simulink model "HDL_DUC"  (R2025a)
settings: Solver=VariableStepAuto  StartTime=0.0  StopTime=sample_period*512*150  RelTol=1e-3
PreLoadFcn:
  | sample_period=1/800e6;
  | dds=80e6; % ddfs frequency
InitFcn:
  | sample_period=1/800e6;
  | dds=80e6; % ddfs frequency
undefined symbols (not defined in the file): A, A2, B, D, PCIN, S, vsva2197, xcvc1902
libraries: hdlBasic x26, hdlDSPIP x5, dspmlti4 x4, simulink x2, vmcUtilities x1
settings Model: Creator=mmi  LastModifiedBy=robg
settings DebuggingCC: ParameterOverflowMsg=warning  UnconnectedInputMsg=warning  UnconnectedOutputMsg=warning  UnconnectedLineMsg=warning
settings HardwareCC: ProdBitPerPointer=32.0  ProdBitPerSizeT=32.0  ProdBitPerPtrDiffT=32.0  ProdLargestAtomicFloat=None  ProdIntDivRoundTo=Undefined  ProdEndianess=Unspecified  ProdWordSize=32.0  ProdHWDeviceType=ASIC/FPGA->ASIC/FPGA  TargetBitPerLong=64.0  TargetBitPerPointer=64.0  TargetBitPerSizeT=64.0  TargetBitPerPtrDiffT=64.0  TargetLongLongMode=on  TargetIntDivRoundTo=Zero  TargetEndianess=LittleEndian  TargetWordSize=64.0  TargetHWDeviceType=Custom Processor->MATLAB Host Computer  ProdEqTarget=off
settings ModelReferenceCC: EnableRefExpFcnMdlSchedulingChecks=on
settings RTWCC: GPUComputeCapability=3.5  DLArmComputeVersion=19.05

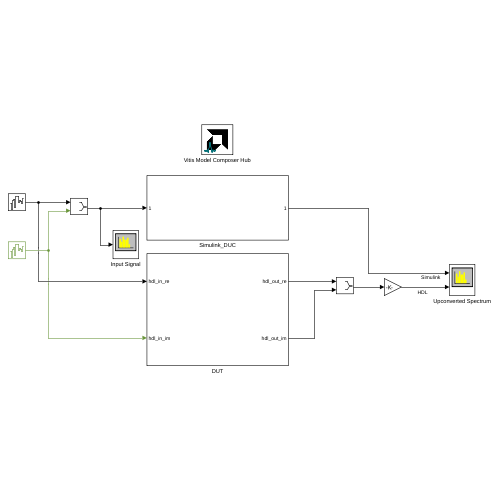
[thumbnail: Simulink's stored preview of the top-level diagram]
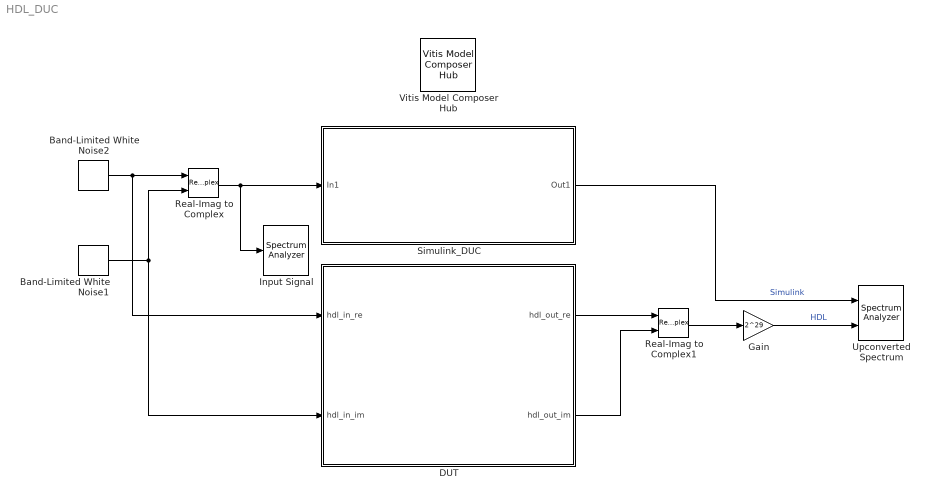
== system HDL_DUC ==
  Band-Limited White Noise1 : simulink/Sources/Band-Limited White Noise  Cov=[0.1]  Ts=sample_period*16  seed=[1]
  Band-Limited White Noise2 : simulink/Sources/Band-Limited White Noise  Cov=[0.1]  Ts=sample_period*16  seed=[2]
  DUT : Subsystem
  Gain : Gain  Gain=2^29  OutDataTypeStr=double
  Input Signal : SpectrumAnalyzer  WindowPosition=[540.000000,419.000000,800.000000,500.000000,]  Visible=on  ScopeFrameLocation=window  Span=50000000  StartFrequency=-25000000  StopFrequency=25000000  YLimits=[22.9484,84.9753]
  Real-Imag to Complex : RealImagToComplex
  Real-Imag to Complex1 : RealImagToComplex
  Simulink_DUC : Subsystem
  Upconverted Spectrum : SpectrumAnalyzer  NumInputPorts=2  WindowPosition=[1096.000000,482.000000,820.000000,457.000000,]  Visible=on  ScopeFrameLocation=window  SampleRate=400000000  AxesScaling=Manual  Span=800000000  StartFrequency=-400000000  StopFrequency=400000000  AveragingMethod=Exponential  YLimits=[63.6592,220.2056]  ShowLegend=on  AllowFFTLengthLessThanSamplesPerUpdate=on
  Vitis Model Composer Hub : vmcUtilities/Vitis Model Composer Hub  Tag=genX  CodeGeneration=off  SubsystemName=DUT  BlockHierPath=HDL_DUC/DUT  CompilationType=HDLCompilation  SubsystemType=HDLNode  ExportTypeV2=IP Catalog  StartColumn=1  NumberOfColumns=1  TargetDirectory=./netlist  exportDesign=on  analyzeDesign=off  validateDesignOnHw=off  ExportType=AI Engines  IpVendor=xilinx.com  IpLibrary=hls  IpVersion=1.0  IpHWLanguage=Verilog  AieCompilerOptions={}  AieSimulatorOptions={}  CreateTestbench=off  TestbenchStackSize=10  RunRtlSim=off  RunCSim=off  RunAieSim=on  enableSimulationTimeout=on  enableGraphIterations=on  AieSimTimeout=50000  AieGraphIterations=-1  RunAieSimProfiling=off  LaunchVitisAnalyzer=on  PlotOutput=off  RunX86Sim=off  X86SimTimeout=10  GenHwImage=off  GenLibadfXo=on  GenHwValidationCode=off  PlatformType=Not Specified  HwSystemType=Baremetal  HwValidationTarget=hw  ProjDevice=xcvc1902-vsva2197-1LP-e-S  ProjDevicePart=xcvc1902-vsva2197-1LP-e-S  AIEType=AIE  SamplePeriod=-1  ClockFrequency=200  DataPathParallelism=1  xilinxfamily=versalaicore  part=xcvc1902  speed=-1LP-e-S  package=vsva2197  directory=./netlist/ip/DUT/src  testbench=off  incr_netlist=off  synthesis_tool=Vivado  clock_wrapper=Clock Enables  dbl_ovrd=According to Block Masks  dcm_input_clock_period=10  sysclk_period=1.25  simulink_period=sample_period  eval_field=0  IPInfoJsonString="{\"DUTSubsystemName\":\"DUT\",\"HDLSubsystem\":{\"SubsystemName\":\"DUT\",\"IPName\":\"HDL_DUC\",\"IPLibrary\":\"VMC\",\"IPVendor\":\"User Company\",\"IPVersion\":\"1.0\",\"TargetDirectory\":\"./netlist\",\"SubsystemDir\":\"./netlist/ip/DUT\",\"FreqHz\":\"800000000\"},\"SubsystemTag\":\"HDLNode\"}"  LogFileName=/proj/xhdhdstaff5/sdegala/Head1/HEAD/VMC_2025_2_July/Examples/HDL/Digital_Filtering/HDL_DUC/netlist/model_composer.log  NThreads=4  IPConfigFile=/tmp/vmctmp-4932002476335468914/HDL_DUC_ipconfig.json
  wires:
  DUT/1(hdl_out_re) -> Real-Imag to Complex1/1
  Simulink_DUC/1(Out1) -> Upconverted Spectrum/1  "Simulink"
  DUT/2(hdl_out_im) -> Real-Imag to Complex1/2
  Real-Imag to Complex1/1 -> Gain/1
  Band-Limited White Noise2/1 -> DUT/1(hdl_in_re), Real-Imag to Complex/1
  Real-Imag to Complex/1 -> Input Signal/1, Simulink_DUC/1(In1)
  Band-Limited White Noise1/1 -> Real-Imag to Complex/2, DUT/2(hdl_in_im)
  Gain/1 -> Upconverted Spectrum/2  "HDL"

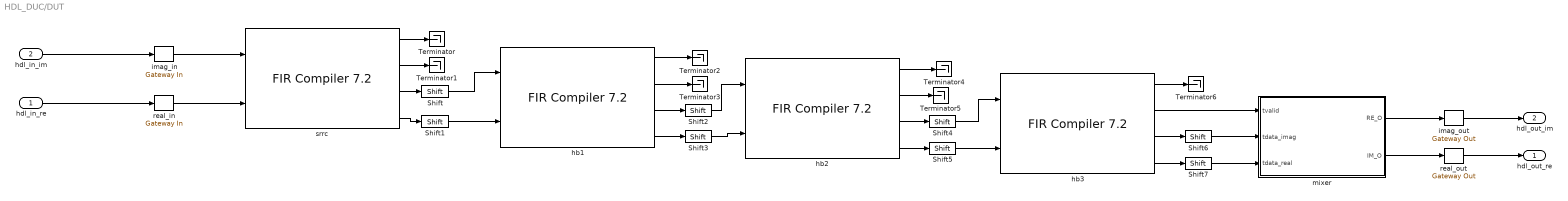
== system HDL_DUC/DUT ==
  hdl_in_re : Inport
  hdl_in_im : Inport  Port=2
  Shift{,1..5} (6 alike) : hdlBasic/Shift  shift_dir=Left  shift_bits=1  en=off  latency=0  precision=Full  arith_type="Signed  (2's comp)"  n_bits=16  bin_pt=14  quantization=Truncate  overflow=Wrap  XmcBlockStatus=1  maskContainerNames=group2  block_type=shift  block_config=sysgen:Shift_config
  Shift6 : hdlBasic/Shift  shift_dir=Left  shift_bits=1  en=off  latency=0  precision=User Defined  arith_type="Signed  (2's comp)"  n_bits=34  bin_pt=0  quantization=Truncate  overflow=Wrap  XmcBlockStatus=1  maskContainerNames=group2  block_type=shift  block_config=sysgen:Shift_config
  Shift7 : hdlBasic/Shift  shift_dir=Left  shift_bits=1  en=off  latency=0  precision=User Defined  arith_type="Signed  (2's comp)"  n_bits=34  bin_pt=0  quantization=Truncate  overflow=Wrap  XmcBlockStatus=1  maskContainerNames=group2  block_type=shift  block_config=sysgen:Shift_config
  Terminator{,1..6} (7 alike) : Terminator
  hb1 : hdlDSPIP/FIR Compiler 7.2   datacoefficienttype=Real  coefficientvector=|  coefficient_sets=1  coefficient_reload=off  filter_type=Interpolation  rate_change_type=Integer  interpolation_rate=2  decimation_rate=1  zero_pack_factor=1  channel_sequence=Basic  number_channels=1  pattern_list='P4-0,P4-1,P4-2,P4-3,P4-4'  number_paths=2  ratespecification=Maximum_Possible  sampleperiod=1  hardwareoversamplingrate=1  coefficient_sign=Signed  quantization=Maximize_Dynamic_Range  coefficient_width=17  bestprecision=on  coefficient_fractional_bits=17  coefficient_structure=Inferred  output_rounding_mode=Truncate_LSBs  output_width=17  filter_architecture=Systolic_Multiply_Accumulate  optimization_goal=Area  optimization_list='None'  data_buffer_type=Automatic  coefficient_buffer_type=Automatic  input_buffer_type=Automatic  output_buffer_type=Automatic  preference_for_other_storage=Automatic  multi_column_support=Automatic  columnconfig='3'  inter_column_pipe_length=4  data_has_tlast=Not_Required  m_data_has_tready=off  s_data_has_fifo=off  s_data_has_tuser=Not_Required  m_data_has_tuser=Not_Required  s_config_sync_mode=On_Vector  s_config_method=Single  num_reload_slots=1  has_aclken=off  has_aresetn=off  reset_data_vector=on  blank_output=off  reset_coeff_vector=off  trim_axipin_name=on  simulation_type=hybrid_sim  simulation_model=sysgen:xfirv7_2_cmodel  data_path_portlist={ 's_axis_data_tdata', 'm_axis_data_tdata' }  passband_min=0.0  passband_max=0.5  stopband_min=0.5  stopband_max=1.0  filter_selection=1  gui_behaviour='Sysgen_GUI'  data_sign=Signed  data_width=16  data_fractional_bits=0  data_tuser_width=1  wrapper_available=true  ip_wrap_arbitrary_binary_point=true  ip_name=FIR Compiler  ip_version=7.2  dsptool_ready=true  ipcore_usecache=true  ipcore_useipmodelcache=true  port_translation_map={ 'aclken' => 'en', 'aresetn' => 'rst' }  run_core_at_system_period=true  ipcore_xco_need_fpga_part=true  ipcore_fpga_part=[]  XmcBlockStatus=1  maskContainerNames=tabcontainer1  block_type=fir_compiler_v7_2  block_config=sysgen:rodinimport_config  block_width=820  block_height=600
      | [-4.347138e-04,
      | 0.000000e+00,
      | 2.889073e-03,
      | 0.000000e+00,
      | -1.100753e-02,
      | 0.000000e+00,
      | 3.178616e-02,
      | 0.000000e+00,
      | -8.312888e-02,
      | 0.000000e+00,
      | 3.098590e-01,
      | 4.999390e-01,
      | 3.098590e-01,
      | 0.000000e+00,
      | -8.312888e-02,
      | 0.000000e+00,
      | 3.178616e-02,
      | 0.000000e+00,
      | -1.100753e-02,
      | 0.000000e+00,
      | 2.889073e-03,
      | 0.000000e+00,
      | -4.347138e-04 
      | ]
  hb2 : hdlDSPIP/FIR Compiler 7.2   datacoefficienttype=Real  coefficientvector=|  coefficient_sets=1  coefficient_reload=off  filter_type=Interpolation  rate_change_type=Integer  interpolation_rate=2  decimation_rate=1  zero_pack_factor=1  channel_sequence=Basic  number_channels=1  pattern_list='P4-0,P4-1,P4-2,P4-3,P4-4'  number_paths=2  ratespecification=Maximum_Possible  sampleperiod=2  hardwareoversamplingrate=1  coefficient_sign=Signed  quantization=Maximize_Dynamic_Range  coefficient_width=17  bestprecision=on  coefficient_fractional_bits=17  coefficient_structure=Inferred  output_rounding_mode=Truncate_LSBs  output_width=17  filter_architecture=Systolic_Multiply_Accumulate  optimization_goal=Area  optimization_list='None'  data_buffer_type=Automatic  coefficient_buffer_type=Automatic  input_buffer_type=Automatic  output_buffer_type=Automatic  preference_for_other_storage=Automatic  multi_column_support=Automatic  columnconfig='2'  inter_column_pipe_length=4  data_has_tlast=Not_Required  m_data_has_tready=off  s_data_has_fifo=off  s_data_has_tuser=Not_Required  m_data_has_tuser=Not_Required  s_config_sync_mode=On_Vector  s_config_method=Single  num_reload_slots=1  has_aclken=off  has_aresetn=off  reset_data_vector=on  blank_output=off  reset_coeff_vector=off  trim_axipin_name=on  simulation_type=hybrid_sim  simulation_model=sysgen:xfirv7_2_cmodel  data_path_portlist={ 's_axis_data_tdata', 'm_axis_data_tdata' }  passband_min=0.0  passband_max=0.5  stopband_min=0.5  stopband_max=1.0  filter_selection=1  gui_behaviour='Sysgen_GUI'  data_sign=Signed  data_width=16  data_fractional_bits=0  data_tuser_width=1  wrapper_available=true  ip_wrap_arbitrary_binary_point=true  ip_name=FIR Compiler  ip_version=7.2  dsptool_ready=true  ipcore_usecache=true  ipcore_useipmodelcache=true  port_translation_map={ 'aclken' => 'en', 'aresetn' => 'rst' }  run_core_at_system_period=true  ipcore_xco_need_fpga_part=true  ipcore_fpga_part=[]  XmcBlockStatus=1  maskContainerNames=tabcontainer1  block_type=fir_compiler_v7_2  block_config=sysgen:rodinimport_config  block_width=820  block_height=600
      | [7.416439e-03,
      | 0.000000e+00,
      | -5.306043e-02,
      | 0.000000e+00,
      | 2.956309e-01,
      | 4.999390e-01,
      | 2.956309e-01,
      | 0.000000e+00,
      | -5.306043e-02,
      | 0.000000e+00,
      | 7.416439e-03 
      | ]
  hb3 : hdlDSPIP/FIR Compiler 7.2   datacoefficienttype=Real  coefficientvector=|  coefficient_sets=1  coefficient_reload=off  filter_type=Interpolation  rate_change_type=Integer  interpolation_rate=2  decimation_rate=1  zero_pack_factor=1  channel_sequence=Basic  number_channels=1  pattern_list='P4-0,P4-1,P4-2,P4-3,P4-4'  number_paths=2  ratespecification=Maximum_Possible  sampleperiod=16  hardwareoversamplingrate=1  coefficient_sign=Signed  quantization=Maximize_Dynamic_Range  coefficient_width=17  bestprecision=on  coefficient_fractional_bits=17  coefficient_structure=Inferred  output_rounding_mode=Truncate_LSBs  output_width=17  filter_architecture=Systolic_Multiply_Accumulate  optimization_goal=Area  optimization_list='None'  data_buffer_type=Automatic  coefficient_buffer_type=Automatic  input_buffer_type=Automatic  output_buffer_type=Automatic  preference_for_other_storage=Automatic  multi_column_support=Automatic  columnconfig='1'  inter_column_pipe_length=4  data_has_tlast=Not_Required  m_data_has_tready=off  s_data_has_fifo=off  s_data_has_tuser=Not_Required  m_data_has_tuser=Not_Required  s_config_sync_mode=On_Vector  s_config_method=Single  num_reload_slots=1  has_aclken=off  has_aresetn=off  reset_data_vector=on  blank_output=off  reset_coeff_vector=off  trim_axipin_name=on  simulation_type=hybrid_sim  simulation_model=sysgen:xfirv7_2_cmodel  data_path_portlist={ 's_axis_data_tdata', 'm_axis_data_tdata' }  passband_min=0.0  passband_max=0.5  stopband_min=0.5  stopband_max=1.0  filter_selection=1  gui_behaviour='Sysgen_GUI'  data_sign=Signed  data_width=16  data_fractional_bits=0  data_tuser_width=1  wrapper_available=true  ip_wrap_arbitrary_binary_point=true  ip_name=FIR Compiler  ip_version=7.2  dsptool_ready=true  ipcore_usecache=true  ipcore_useipmodelcache=true  port_translation_map={ 'aclken' => 'en', 'aresetn' => 'rst' }  run_core_at_system_period=true  ipcore_xco_need_fpga_part=true  ipcore_fpga_part=[]  XmcBlockStatus=1  maskContainerNames=tabcontainer1  block_type=fir_compiler_v7_2  block_config=sysgen:rodinimport_config  block_width=820  block_height=600
      | [-3.216511e-02,
      | 0.000000e+00,
      | 2.821170e-01,
      | 4.999390e-01,
      | 2.821170e-01,
      | 0.000000e+00,
      | -3.216511e-02]
  imag_in : hdlBasic/Gateway In  gui_display_data_type=Fixed-point  arith_type=Signed (2's comp)  n_bits=17  bin_pt=14  preci_type=Single  exp_width=8  frac_width=24  rows=1  columns=1  quantization=Truncate  overflow=Wrap  period=sample_period*16  UseAsADC=off  ADCChannel='1'  interface=None  automatic_assignment=on  address_offset=hex2dec('00')  intf_name=''  intf_description=''  default_value=0  timing_constraint=None  locs_specified=off  LOCs={}  io_standard={}  inherit_from_input=off  hdl_port=on  XmcBlockStatus=1  maskContainerNames=group4  block_type=gatewayin  block_config=sysgen:gateway_in_config  block_width_w=590  block_height_w=620  block_width=640  block_height=850
  imag_out : hdlBasic/Gateway Out  inherit_from_input=off  bool_to_boolean=off  hdl_port=on  rows=1  columns=1  UseAsDAC=off  DACChannel='1'  interface=None  automatic_assignment=on  address_offset=hex2dec('00')  intf_name=''  intf_description=''  timing_constraint=None  locs_specified=off  LOCs={}  io_standard={}  XmcBlockStatus=1  maskContainerNames=group4  block_type=gatewayout  block_config=sysgen:gateway_out_config  block_width_w=590  block_height_w=620  block_width=620  block_height=750
  mixer : Subsystem
  real_in : hdlBasic/Gateway In  gui_display_data_type=Fixed-point  arith_type=Signed (2's comp)  n_bits=17  bin_pt=14  preci_type=Single  exp_width=8  frac_width=24  rows=1  columns=1  quantization=Truncate  overflow=Wrap  period=sample_period*16  UseAsADC=off  ADCChannel='1'  interface=None  automatic_assignment=on  address_offset=hex2dec('00')  intf_name=''  intf_description=''  default_value=0  timing_constraint=None  locs_specified=off  LOCs={}  io_standard={}  inherit_from_input=off  hdl_port=on  XmcBlockStatus=1  maskContainerNames=group4  block_type=gatewayin  block_config=sysgen:gateway_in_config  block_width_w=590  block_height_w=620  block_width=640  block_height=850
  real_out : hdlBasic/Gateway Out  inherit_from_input=off  bool_to_boolean=off  hdl_port=on  rows=1  columns=1  UseAsDAC=off  DACChannel='1'  interface=None  automatic_assignment=on  address_offset=hex2dec('00')  intf_name=''  intf_description=''  timing_constraint=None  locs_specified=off  LOCs={}  io_standard={}  XmcBlockStatus=1  maskContainerNames=group4  block_type=gatewayout  block_config=sysgen:gateway_out_config  block_width_w=590  block_height_w=620  block_width=620  block_height=750
  srrc : hdlDSPIP/FIR Compiler 7.2   datacoefficienttype=Real  coefficientvector=|  coefficient_sets=1  coefficient_reload=off  filter_type=Interpolation  rate_change_type=Integer  interpolation_rate=2  decimation_rate=1  zero_pack_factor=1  channel_sequence=Basic  number_channels=1  pattern_list='P4-0,P4-1,P4-2,P4-3,P4-4'  number_paths=2  ratespecification=Maximum_Possible  sampleperiod=1  hardwareoversamplingrate=1  coefficient_sign=Signed  quantization=Maximize_Dynamic_Range  coefficient_width=17  bestprecision=on  coefficient_fractional_bits=16  coefficient_structure=Inferred  output_rounding_mode=Truncate_LSBs  output_width=17  filter_architecture=Systolic_Multiply_Accumulate  optimization_goal=Area  optimization_list='None'  data_buffer_type=Automatic  coefficient_buffer_type=Automatic  input_buffer_type=Automatic  output_buffer_type=Automatic  preference_for_other_storage=Automatic  multi_column_support=Automatic  columnconfig='17'  inter_column_pipe_length=4  data_has_tlast=Not_Required  m_data_has_tready=off  s_data_has_fifo=off  s_data_has_tuser=Not_Required  m_data_has_tuser=Not_Required  s_config_sync_mode=On_Vector  s_config_method=Single  num_reload_slots=1  has_aclken=off  has_aresetn=off  reset_data_vector=on  blank_output=off  reset_coeff_vector=off  trim_axipin_name=on  simulation_type=hybrid_sim  simulation_model=sysgen:xfirv7_2_cmodel  data_path_portlist={ 's_axis_data_tdata', 'm_axis_data_tdata' }  passband_min=0.0  passband_max=0.5  stopband_min=0.5  stopband_max=1.0  filter_selection=1  gui_behaviour='Sysgen_GUI'  data_sign=Signed  data_width=16  data_fractional_bits=0  data_tuser_width=1  wrapper_available=true  ip_wrap_arbitrary_binary_point=true  ip_name=FIR Compiler  ip_version=7.2  dsptool_ready=true  ipcore_usecache=true  ipcore_useipmodelcache=true  port_translation_map={ 'aclken' => 'en', 'aresetn' => 'rst' }  run_core_at_system_period=true  ipcore_xco_need_fpga_part=true  ipcore_fpga_part=[]  XmcBlockStatus=1  maskContainerNames=tabcontainer1  block_type=fir_compiler_v7_2  block_config=sysgen:rodinimport_config  block_width=820  block_height=600
      | [8.538552e-06,
      | 4.669178e-07,
      | -3.697474e-05,
      | 3.052152e-06,
      | 1.093230e-04,
      | -2.416268e-05,
      | -2.637924e-04,
      | 9.271878e-05,
      | 5.516021e-04,
      | -2.673026e-04,
      | -1.035981e-03,
      | 6.447576e-04,
      | 1.781800e-03,
      | -1.374126e-03,
      | -2.845114e-03,
      | 2.666081e-03,
      | 4.255749e-03,
      | -4.808402e-03,
      | -6.004074e-03,
      | 8.189170e-03,
      | 8.028184e-03,
      | -1.336089e-02,
      | -1.021252e-02,
      | 2.121003e-02,
      | 1.239342e-02,
      | -3.346770e-02,
      | -1.437864e-02,
      | 5.450117e-02,
      | 1.597204e-02,
      | -1.003560e-01,
      | -1.700502e-02,
      | 3.163505e-01,
      | 5.173627e-01,
      | 3.163505e-01,
      | -1.700502e-02,
      | -1.003560e-01,
      | 1.597204e-02,
      | 5.450117e-02,
      | -1.437864e-02,
      | -3.346770e-02,
      | 1.239342e-02,
      | 2.121003e-02,
      | -1.021252e-02,
      | -1.336089e-02,
      | 8.028184e-03,
      | 8.189170e-03,
      | -6.004074e-03,
      | -4.808402e-03,
      | 4.255749e-03,
      | 2.666081e-03,
      | -2.845114e-03,
      | -1.374126e-03,
      | 1.781800e-03,
      | 6.447576e-04,
      | -1.035981e-03,
      | -2.673026e-04,
      | 5.516021e-04,
      | 9.271878e-05,
      | -2.637924e-04,
      | -2.416268e-05,
      | 1.093230e-04,
      | 3.052152e-06,
      | -3.697474e-05,
      | 4.669178e-07,
      | 8.538552e-06]
  hdl_out_re : Outport
  hdl_out_im : Outport  Port=2
  wires:
  hb2/2 -> Terminator5/1
  Shift/1 -> hb1/1
  Shift3/1 -> hb2/2
  srrc/2 -> Terminator1/1
  srrc/3 -> Shift/1
  real_out/1 -> hdl_out_re/1
  Shift5/1 -> hb3/2
  hb3/1 -> Terminator6/1
  srrc/1 -> Terminator/1
  hb1/3 -> Shift2/1
  srrc/4 -> Shift1/1
  hdl_in_re/1 -> real_in/1
  hb2/3 -> Shift4/1
  hb3/4 -> Shift7/1
  imag_out/1 -> hdl_out_im/1
  hb2/1 -> Terminator4/1
  hdl_in_im/1 -> imag_in/1
  hb1/1 -> Terminator2/1
  hb1/4 -> Shift3/1
  hb1/2 -> Terminator3/1
  real_in/1 -> srrc/2
  hb3/3 -> Shift6/1
  Shift1/1 -> hb1/2
  imag_in/1 -> srrc/1
  Shift2/1 -> hb2/1
  Shift4/1 -> hb3/1
  hb2/4 -> Shift5/1
  mixer/1(RE_O) -> imag_out/1
  mixer/2(IM_O) -> real_out/1
  hb3/2 -> mixer/1(tvalid)
  Shift6/1 -> mixer/2(tdata_imag)
  Shift7/1 -> mixer/3(tdata_real)

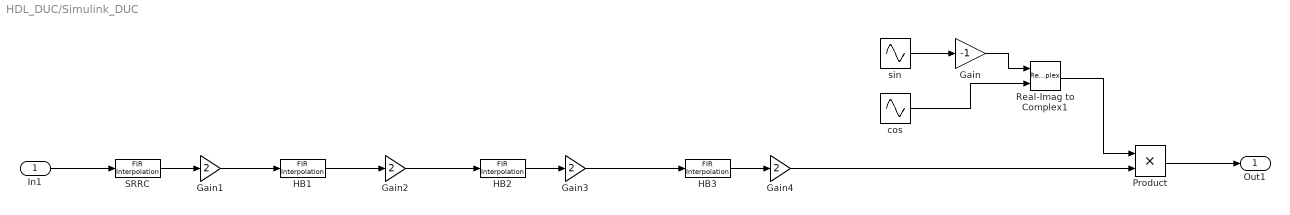
== system HDL_DUC/Simulink_DUC ==
  In1 : Inport
  Gain : Gain  Gain=-1
  Gain{1..4} (4 alike) : Gain  Gain=2
  HB1 : dspmlti4/FIR Interpolation  FilterSource=Dialog parameters  PrivateCoeffs=0  h=|  L=2  FilterObject=FINTERP  framing=Allow multirate processing  outputBufInitCond=0  roundingMode=Floor  overflowMode=off  firstCoeffDataTypeStr=Inherit: Same word length as input  firstCoeffMin=[]  firstCoeffMax=[]  firstCoeffLastDataTypeStr=Inherit: Same word length as input  outputDataTypeStr=Inherit: Same as accumulator  outputMin=[]  outputMax=[]  outputLastDataTypeStr=Inherit: Same as accumulator
      | [-4.347138e-04,
      | 0.000000e+00,
      | 2.889073e-03,
      | 0.000000e+00,
      | -1.100753e-02,
      | 0.000000e+00,
      | 3.178616e-02,
      | 0.000000e+00,
      | -8.312888e-02,
      | 0.000000e+00,
      | 3.098590e-01,
      | 4.999390e-01,
      | 3.098590e-01,
      | 0.000000e+00,
      | -8.312888e-02,
      | 0.000000e+00,
      | 3.178616e-02,
      | 0.000000e+00,
      | -1.100753e-02,
      | 0.000000e+00,
      | 2.889073e-03,
      | 0.000000e+00,
      | -4.347138e-04 
      | ]
  HB2 : dspmlti4/FIR Interpolation  FilterSource=Dialog parameters  PrivateCoeffs=0  h=|  L=2  FilterObject=FINTERP  framing=Allow multirate processing  outputBufInitCond=0  roundingMode=Floor  overflowMode=off  firstCoeffDataTypeStr=Inherit: Same word length as input  firstCoeffMin=[]  firstCoeffMax=[]  firstCoeffLastDataTypeStr=Inherit: Same word length as input  outputDataTypeStr=Inherit: Same as accumulator  outputMin=[]  outputMax=[]  outputLastDataTypeStr=Inherit: Same as accumulator
      | [7.416439e-03,
      | 0.000000e+00,
      | -5.306043e-02,
      | 0.000000e+00,
      | 2.956309e-01,
      | 4.999390e-01,
      | 2.956309e-01,
      | 0.000000e+00,
      | -5.306043e-02,
      | 0.000000e+00,
      | 7.416439e-03 
      | ]
  HB3 : dspmlti4/FIR Interpolation  FilterSource=Dialog parameters  PrivateCoeffs=0  h=|  L=2  FilterObject=FINTERP  framing=Allow multirate processing  outputBufInitCond=0  roundingMode=Floor  overflowMode=off  firstCoeffDataTypeStr=Inherit: Same word length as input  firstCoeffMin=[]  firstCoeffMax=[]  firstCoeffLastDataTypeStr=Inherit: Same word length as input  outputDataTypeStr=Inherit: Same as accumulator  outputMin=[]  outputMax=[]  outputLastDataTypeStr=Inherit: Same as accumulator
      | [-3.216511e-02,
      | 0.000000e+00,
      | 2.821170e-01,
      | 4.999390e-01,
      | 2.821170e-01,
      | 0.000000e+00,
      | -3.216511e-02]
  Product : Product
  Real-Imag to Complex1 : RealImagToComplex
  SRRC : dspmlti4/FIR Interpolation  FilterSource=Dialog parameters  PrivateCoeffs=0  h=|  L=2  FilterObject=FINTERP  framing=Allow multirate processing  outputBufInitCond=0  roundingMode=Floor  overflowMode=off  firstCoeffDataTypeStr=Inherit: Same word length as input  firstCoeffMin=[]  firstCoeffMax=[]  firstCoeffLastDataTypeStr=Inherit: Same word length as input  outputDataTypeStr=Inherit: Same as accumulator  outputMin=[]  outputMax=[]  outputLastDataTypeStr=Inherit: Same as accumulator
      | [8.538552e-06,
      | 4.669178e-07,
      | -3.697474e-05,
      | 3.052152e-06,
      | 1.093230e-04,
      | -2.416268e-05,
      | -2.637924e-04,
      | 9.271878e-05,
      | 5.516021e-04,
      | -2.673026e-04,
      | -1.035981e-03,
      | 6.447576e-04,
      | 1.781800e-03,
      | -1.374126e-03,
      | -2.845114e-03,
      | 2.666081e-03,
      | 4.255749e-03,
      | -4.808402e-03,
      | -6.004074e-03,
      | 8.189170e-03,
      | 8.028184e-03,
      | -1.336089e-02,
      | -1.021252e-02,
      | 2.121003e-02,
      | 1.239342e-02,
      | -3.346770e-02,
      | -1.437864e-02,
      | 5.450117e-02,
      | 1.597204e-02,
      | -1.003560e-01,
      | -1.700502e-02,
      | 3.163505e-01,
      | 5.173627e-01,
      | 3.163505e-01,
      | -1.700502e-02,
      | -1.003560e-01,
      | 1.597204e-02,
      | 5.450117e-02,
      | -1.437864e-02,
      | -3.346770e-02,
      | 1.239342e-02,
      | 2.121003e-02,
      | -1.021252e-02,
      | -1.336089e-02,
      | 8.028184e-03,
      | 8.189170e-03,
      | -6.004074e-03,
      | -4.808402e-03,
      | 4.255749e-03,
      | 2.666081e-03,
      | -2.845114e-03,
      | -1.374126e-03,
      | 1.781800e-03,
      | 6.447576e-04,
      | -1.035981e-03,
      | -2.673026e-04,
      | 5.516021e-04,
      | 9.271878e-05,
      | -2.637924e-04,
      | -2.416268e-05,
      | 1.093230e-04,
      | 3.052152e-06,
      | -3.697474e-05,
      | 4.669178e-07,
      | 8.538552e-06]
  cos : Sin  Amplitude=2^8  Frequency=80e6*2*pi  Phase=pi/2  SampleTime=sample_period  VectorParams1D=off
  sin : Sin  Amplitude=2^8  Frequency=80e6*2*pi  SampleTime=sample_period  VectorParams1D=off
  Out1 : Outport
  wires:
  sin/1 -> Gain/1
  Gain1/1 -> HB1/1
  SRRC/1 -> Gain1/1
  HB2/1 -> Gain3/1
  Gain4/1 -> Product/2
  Gain2/1 -> HB2/1
  Real-Imag to Complex1/1 -> Product/1
  Gain3/1 -> HB3/1
  HB1/1 -> Gain2/1
  HB3/1 -> Gain4/1
  Product/1 -> Out1/1
  In1/1 -> SRRC/1
  cos/1 -> Real-Imag to Complex1/2
  Gain/1 -> Real-Imag to Complex1/1

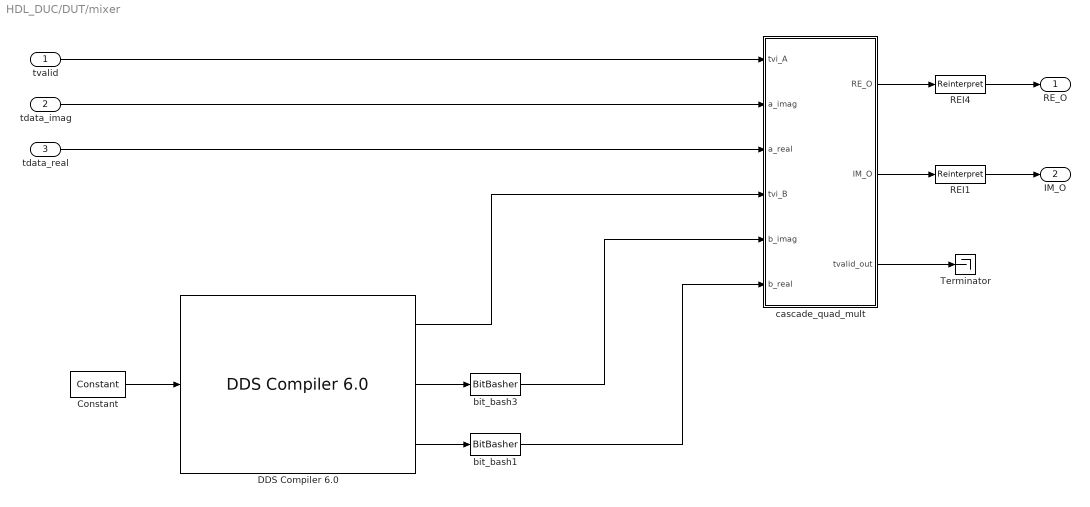
== system HDL_DUC/DUT/mixer ==
  tvalid : Inport
  tdata_imag : Inport  Port=2
  tdata_real : Inport  Port=3
  Constant : hdlBasic/Constant  const=1  gui_display_data_type=Boolean  arith_type=Boolean  n_bits=16  bin_pt=14  preci_type=Single  exp_width=8  frac_width=24  explicit_period=off  period=1  XmcBlockStatus=1  maskContainerNames=tabcontainer1  block_type=constant  block_config=sysgen:Constant_config
  DDS Compiler 6.0 : hdlDSPIP/DDS Compiler 6.0   partspresent=Phase_Generator_and_SIN_COS_LUT  dds_clock_rate=(1/sample_period)/1e6  channels=1  mode_of_operation=Standard  output_type=Integer  modulus=9  parameter_entry=System_Parameters  spurious_free_dynamic_range=85.00000000  frequency_resolution=0.07000000  noise_shaping=Phase_Dithering  phase_width=33  output_width=15  output_selection=Sine_and_Cosine  negative_sine=on  negative_cosine=off  amplitude_mode=Full_Range  memory_type=Auto  optimization_goal=Auto  dsp48_use=Minimal  resync=off  latency_configuration=Auto  latency=1  has_phase_out=off  has_aclken=off  has_aresetn=off  explicit_period=off  period=1  data_has_tlast=Not_Required  has_tready=on  s_phase_has_tuser=Not_Required  m_data_has_tuser=Not_Required  m_phase_has_tuser=Not_Required  s_phase_tuser_width=1  output_form=Twos_Complement  s_config_sync_mode=On_Vector  phase_increment=Fixed  output_frequency1=80  output_frequency2=0  output_frequency3=0  output_frequency4=0  output_frequency5=0  output_frequency6=0  output_frequency7=0  output_frequency8=0  output_frequency9=0  output_frequency10=0  output_frequency11=0  output_frequency12=0  output_frequency13=0  output_frequency14=0  output_frequency15=0  output_frequency16=0  pinc1='1100110011001100110011001100110'  pinc2='0'  pinc3='0'  pinc4='0'  pinc5='0'  pinc6='0'  pinc7='0'  pinc8='0'  pinc9='0'  pinc10='0'  pinc11='0'  pinc12='0'  pinc13='0'  pinc14='0'  pinc15='0'  pinc16='0'  phase_offset=None  phase_offset_angles1=0  phase_offset_angles2=0  phase_offset_angles3=0  phase_offset_angles4=0  phase_offset_angles5=0  phase_offset_angles6=0  phase_offset_angles7=0  phase_offset_angles8=0  phase_offset_angles9=0  phase_offset_angles10=0  phase_offset_angles11=0  phase_offset_angles12=0  phase_offset_angles13=0  phase_offset_angles14=0  phase_offset_angles15=0  phase_offset_angles16=0  poff1='0'  poff2='0'  poff3='0'  poff4='0'  poff5='0'  poff6='0'  poff7='0'  poff8='0'  poff9='0'  poff10='0'  poff11='0'  poff12='0'  poff13='0'  poff14='0'  poff15='0'  poff16='0'  trim_axipin_name=on  simulation_type=hybrid_sim  simulation_model=sysgen:xddsv6_0_cmodel  data_path_portlist={ 's_axis_config_tdata_poff', 's_axis_config_tdata_chan0_poff', 's_axis_config_tdata_pinc', 's_axis_config_tdata_chan0_pinc', 's_axis_phase_tdata_resync', 's_axis_phase_tdata_chan0_resync', 's_axis_phase_tdata_poff', 's_axis_phase_tdata_chan0_poff', 's_axis_phase_tdata_pinc', 's_axis_phase_tdata_chan0_pinc', 's_axis_phase_tdata_phase_in', 'm_axis_data_tdata_sine', 'm_axis_data_tdata_chan0_sine', 'm_axis_data_tdata_cosine', 'm_axis_data_tdata_chan0_cosine', 'm_axis_phase_tdata_phase_out', 'm_axis_phase_tdata_chan0_phase_out'}  por_mode=false  gui_behaviour=Sysgen  ip_name=DDS Compiler  ip_version=6.0  dsptool_ready=true  wrapper_available=true  port_translation_map={ 'aclken' => 'en', 'aresetn' => 'rst' }  ipcore_usecache=true  ipcore_useipmodelcache=true  ipcore_xco_need_fpga_part=true  ipcore_fpga_part=[]  ipcore_verbose=false  XmcBlockStatus=1  maskContainerNames=tabcontainer1  block_type=dds_compiler_v6_0  block_config=sysgen:rodinimport_config  block_width=760
  REI1 : hdlBasic/Reinterpret  force_arith_type=on  arith_type="Signed  (2's comp)"  force_bin_pt=on  bin_pt=26  XmcBlockStatus=1  maskContainerNames=group1  block_type=reinterpret  block_config=sysgen:Reinterpret_config
  REI4 : hdlBasic/Reinterpret  force_arith_type=on  arith_type="Signed  (2's comp)"  force_bin_pt=on  bin_pt=26  XmcBlockStatus=1  maskContainerNames=group1  block_type=reinterpret  block_config=sysgen:Reinterpret_config
  Terminator : Terminator
  bit_bash1 : hdlBasic/BitBasher  bitexpr=ao={ 9{ain[14]} , ain[14:0] }; % sign extend to 24 bit data  display_expr=off  sr_1=ao  arith_type1="Signed  (2's comp)"  bin_pt1=0  sr_2=b_dsp48  arith_type2="Signed  (2's comp)"  bin_pt2=0  sr_3=p2  arith_type3=Unsigned  bin_pt3=0  sr_4=4  arith_type4=Unsigned  bin_pt4=0  XmcBlockStatus=1  maskContainerNames=group1  block_type=bitbasher  block_config=sysgen:BitBasher_config
  bit_bash3 : hdlBasic/BitBasher  bitexpr=ao={ 9{ain[14]} , ain[14:0] }; % sign extend to 24 bit data  display_expr=off  sr_1=ao  arith_type1="Signed  (2's comp)"  bin_pt1=0  sr_2=b_dsp48  arith_type2="Signed  (2's comp)"  bin_pt2=0  sr_3=p2  arith_type3=Unsigned  bin_pt3=0  sr_4=4  arith_type4=Unsigned  bin_pt4=0  XmcBlockStatus=1  maskContainerNames=group1  block_type=bitbasher  block_config=sysgen:BitBasher_config
  cascade_quad_mult : Subsystem
  RE_O : Outport
  IM_O : Outport  Port=2
  wires:
  DDS Compiler 6.0/1 -> cascade_quad_mult/4(tvi_B)
  Constant/1 -> DDS Compiler 6.0/1
  DDS Compiler 6.0/2 -> bit_bash3/1
  DDS Compiler 6.0/3 -> bit_bash1/1
  tvalid/1 -> cascade_quad_mult/1(tvi_A)
  cascade_quad_mult/1(RE_O) -> REI4/1
  tdata_imag/1 -> cascade_quad_mult/2(a_imag)
  tdata_real/1 -> cascade_quad_mult/3(a_real)
  cascade_quad_mult/3(tvalid_out) -> Terminator/1
  cascade_quad_mult/2(IM_O) -> REI1/1
  REI4/1 -> RE_O/1
  REI1/1 -> IM_O/1
  bit_bash3/1 -> cascade_quad_mult/5(b_imag)
  bit_bash1/1 -> cascade_quad_mult/6(b_real)

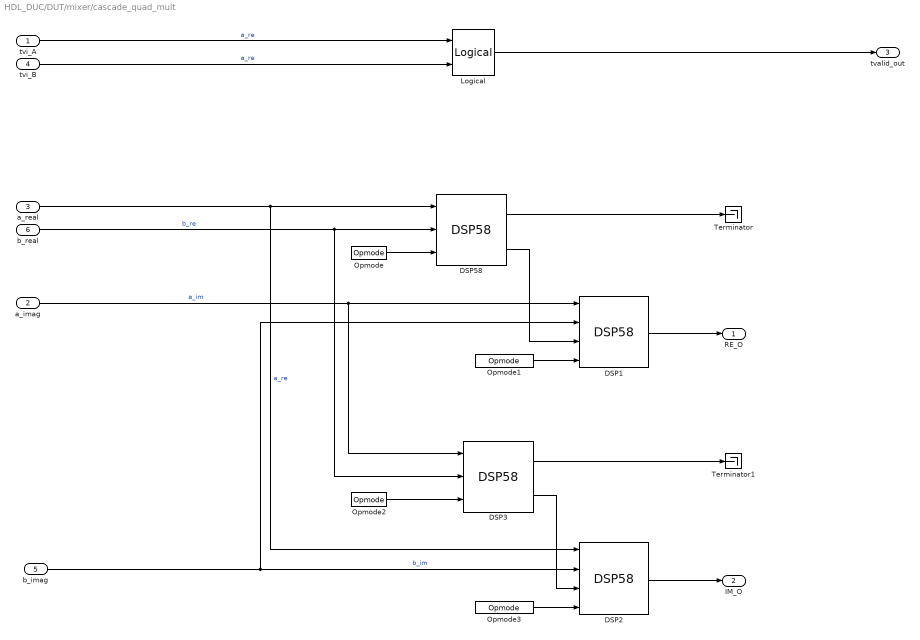
== system HDL_DUC/DUT/mixer/cascade_quad_mult ==
  tvi_A : Inport
  a_imag : Inport  Port=2
  a_real : Inport  Port=3
  tvi_B : Inport  Port=4
  b_imag : Inport  Port=5
  b_real : Inport  Port=6
  DSP1 : hdlBasic/DSP58   use_a=Direct from a port  use_b=Direct from b port  addsub_mode=One 58-bit Unit  dsp_mode=27x24 fixed point  xl_useadderonly=off  xl_dynamicmult=off  preaddinsel=A  amultsel=A  bmultsel=B  enable_d=off  reset_preg=off  auto_reset_pr=RESET  pattern_from_creg=Pattern Input from c port  pattern='000000000000000'  mask_from_creg=Mask Input from c port  pattern_mask='000000000000000'  rnd='000000000000000'  widexor=off  xormode=XOR12  use_op=on  use_creg=off  rst_all=off  en_all=off  use_pcin=on  use_carrycascin=off  use_multsignin=off  use_carryout=off  use_patterndetect=off  use_patternbdetect=off  use_overflow=off  use_underflow=off  use_acout=off  use_bcout=off  use_pcout=off  use_multsignout=off  use_carrycascout=off  pipeline_a=2  pipeline_b=2  pipeline_acout=1  pipeline_bcout=1  pipeline_c=on  pipeline_p=on  pipeline_mult=on  pipeline_opmode=on  pipeline_alumode=on  pipeline_carryin=on  pipeline_carryinsel=on  dreg=off  adreg=off  register_inmode=off  rst_a=off  rst_b=off  rst_c=off  rst_mult=off  rst_p=off  rst_carry_in=off  rst_alumode=off  rst_ctrl=off  reset_port_d=off  reset_port_inmode=off  en_a1=off  en_a2=off  en_b1=off  en_b2=off  en_c=off  en_mult=off  en_p=off  en_carry_in=off  en_alumode=off  en_multcarryin=off  en_ctrl=off  enable_port_regd=off  enable_port_regad=off  enable_port_reginmode=off  alumode_inverted=off  alumode_inverted_value='0000'  is_carryin_inverted=off  inmode_inverted=off  inmode_inverted_value='00000'  negate_inverted=off  negate_inverted_value='000'  opmode_inverted=off  opmode_inverted_value='000000000'  is_rstallcarryin_inverted=off  is_rstalumode_inverted=off  is_rsta_inverted=off  is_rstb_inverted=off  is_rstc_inverted=off  is_rstd_inverted=off  is_rstctrl_inverted=off  is_rstinmode_inverted=off  is_rstm_inverted=off  is_rstp_inverted=off  use_synth_model=off  simulation_type=fast_sim  is_clk_inverted=false  reset_mode=SYNC  XmcBlockStatus=1  maskContainerNames=tabcontainer1  block_type=dsp58  block_config=sysgen:DSP58_config  block_height=1080  block_width=800
  DSP2 : hdlBasic/DSP58   use_a=Direct from a port  use_b=Direct from b port  addsub_mode=One 58-bit Unit  dsp_mode=27x24 fixed point  xl_useadderonly=off  xl_dynamicmult=off  preaddinsel=A  amultsel=A  bmultsel=B  enable_d=off  reset_preg=off  auto_reset_pr=RESET  pattern_from_creg=Pattern Input from c port  pattern='000000000000000'  mask_from_creg=Mask Input from c port  pattern_mask='000000000000000'  rnd='000000000000000'  widexor=off  xormode=XOR12  use_op=on  use_creg=off  rst_all=off  en_all=off  use_pcin=on  use_carrycascin=off  use_multsignin=off  use_carryout=off  use_patterndetect=off  use_patternbdetect=off  use_overflow=off  use_underflow=off  use_acout=off  use_bcout=off  use_pcout=off  use_multsignout=off  use_carrycascout=off  pipeline_a=2  pipeline_b=2  pipeline_acout=1  pipeline_bcout=1  pipeline_c=on  pipeline_p=on  pipeline_mult=on  pipeline_opmode=on  pipeline_alumode=on  pipeline_carryin=on  pipeline_carryinsel=on  dreg=off  adreg=off  register_inmode=off  rst_a=off  rst_b=off  rst_c=off  rst_mult=off  rst_p=off  rst_carry_in=off  rst_alumode=off  rst_ctrl=off  reset_port_d=off  reset_port_inmode=off  en_a1=off  en_a2=off  en_b1=off  en_b2=off  en_c=off  en_mult=off  en_p=off  en_carry_in=off  en_alumode=off  en_multcarryin=off  en_ctrl=off  enable_port_regd=off  enable_port_regad=off  enable_port_reginmode=off  alumode_inverted=off  alumode_inverted_value='0000'  is_carryin_inverted=off  inmode_inverted=off  inmode_inverted_value='00000'  negate_inverted=off  negate_inverted_value='000'  opmode_inverted=off  opmode_inverted_value='000000000'  is_rstallcarryin_inverted=off  is_rstalumode_inverted=off  is_rsta_inverted=off  is_rstb_inverted=off  is_rstc_inverted=off  is_rstd_inverted=off  is_rstctrl_inverted=off  is_rstinmode_inverted=off  is_rstm_inverted=off  is_rstp_inverted=off  use_synth_model=off  simulation_type=fast_sim  is_clk_inverted=false  reset_mode=SYNC  XmcBlockStatus=1  maskContainerNames=tabcontainer1  block_type=dsp58  block_config=sysgen:DSP58_config  block_height=1080  block_width=800
  DSP3 : hdlBasic/DSP58   use_a=Direct from a port  use_b=Direct from b port  addsub_mode=One 58-bit Unit  dsp_mode=27x24 fixed point  xl_useadderonly=off  xl_dynamicmult=off  preaddinsel=A  amultsel=A  bmultsel=B  enable_d=off  reset_preg=off  auto_reset_pr=RESET  pattern_from_creg=Pattern Input from c port  pattern='000000000000000'  mask_from_creg=Mask Input from c port  pattern_mask='000000000000000'  rnd='000000000000000'  widexor=off  xormode=XOR12  use_op=on  use_creg=off  rst_all=off  en_all=off  use_pcin=off  use_carrycascin=off  use_multsignin=off  use_carryout=off  use_patterndetect=off  use_patternbdetect=off  use_overflow=off  use_underflow=off  use_acout=off  use_bcout=off  use_pcout=on  use_multsignout=off  use_carrycascout=off  pipeline_a=1  pipeline_b=1  pipeline_acout=1  pipeline_bcout=1  pipeline_c=on  pipeline_p=on  pipeline_mult=on  pipeline_opmode=on  pipeline_alumode=on  pipeline_carryin=on  pipeline_carryinsel=on  dreg=off  adreg=off  register_inmode=off  rst_a=off  rst_b=off  rst_c=off  rst_mult=off  rst_p=off  rst_carry_in=off  rst_alumode=off  rst_ctrl=off  reset_port_d=off  reset_port_inmode=off  en_a1=off  en_a2=off  en_b1=off  en_b2=off  en_c=off  en_mult=off  en_p=off  en_carry_in=off  en_alumode=off  en_multcarryin=off  en_ctrl=off  enable_port_regd=off  enable_port_regad=off  enable_port_reginmode=off  alumode_inverted=off  alumode_inverted_value='0000'  is_carryin_inverted=off  inmode_inverted=off  inmode_inverted_value='00000'  negate_inverted=off  negate_inverted_value='000'  opmode_inverted=off  opmode_inverted_value='000000000'  is_rstallcarryin_inverted=off  is_rstalumode_inverted=off  is_rsta_inverted=off  is_rstb_inverted=off  is_rstc_inverted=off  is_rstd_inverted=off  is_rstctrl_inverted=off  is_rstinmode_inverted=off  is_rstm_inverted=off  is_rstp_inverted=off  use_synth_model=off  simulation_type=fast_sim  is_clk_inverted=false  reset_mode=SYNC  XmcBlockStatus=1  maskContainerNames=tabcontainer1  block_type=dsp58  block_config=sysgen:DSP58_config  block_height=1080  block_width=800
  DSP58 : hdlBasic/DSP58   use_a=Direct from a port  use_b=Direct from b port  addsub_mode=One 58-bit Unit  dsp_mode=27x24 fixed point  xl_useadderonly=off  xl_dynamicmult=off  preaddinsel=A  amultsel=A  bmultsel=B  enable_d=off  reset_preg=off  auto_reset_pr=RESET  pattern_from_creg=Pattern Input from c port  pattern='000000000000000'  mask_from_creg=Mask Input from c port  pattern_mask='000000000000000'  rnd='000000000000000'  widexor=off  xormode=XOR12  use_op=on  use_creg=off  rst_all=off  en_all=off  use_pcin=off  use_carrycascin=off  use_multsignin=off  use_carryout=off  use_patterndetect=off  use_patternbdetect=off  use_overflow=off  use_underflow=off  use_acout=off  use_bcout=off  use_pcout=on  use_multsignout=off  use_carrycascout=off  pipeline_a=1  pipeline_b=1  pipeline_acout=1  pipeline_bcout=1  pipeline_c=on  pipeline_p=on  pipeline_mult=on  pipeline_opmode=on  pipeline_alumode=on  pipeline_carryin=on  pipeline_carryinsel=on  dreg=off  adreg=off  register_inmode=off  rst_a=off  rst_b=off  rst_c=off  rst_mult=off  rst_p=off  rst_carry_in=off  rst_alumode=off  rst_ctrl=off  reset_port_d=off  reset_port_inmode=off  en_a1=off  en_a2=off  en_b1=off  en_b2=off  en_c=off  en_mult=off  en_p=off  en_carry_in=off  en_alumode=off  en_multcarryin=off  en_ctrl=off  enable_port_regd=off  enable_port_regad=off  enable_port_reginmode=off  alumode_inverted=off  alumode_inverted_value='0000'  is_carryin_inverted=off  inmode_inverted=off  inmode_inverted_value='00000'  negate_inverted=off  negate_inverted_value='000'  opmode_inverted=off  opmode_inverted_value='000000000'  is_rstallcarryin_inverted=off  is_rstalumode_inverted=off  is_rsta_inverted=off  is_rstb_inverted=off  is_rstc_inverted=off  is_rstd_inverted=off  is_rstctrl_inverted=off  is_rstinmode_inverted=off  is_rstm_inverted=off  is_rstp_inverted=off  use_synth_model=off  simulation_type=fast_sim  is_clk_inverted=false  reset_mode=SYNC  XmcBlockStatus=1  maskContainerNames=tabcontainer1  block_type=dsp58  block_config=sysgen:DSP58_config  block_height=1080  block_width=800
  Logical : hdlBasic/Logical  logical_function=AND  inputs=2  en=off  latency=4  precision=Full  arith_type=Unsigned  n_bits=16  bin_pt=0  align_bp=on  overflow=[]  quantization=[]  XmcBlockStatus=1  maskContainerNames=tabcontainer1  block_type=logical  block_config=sysgen:Logical_config
  Opmode : hdlBasic/Opmode  device=DSP58  equ=P=(A*B)  operation=A * B  inmode_0_3=D+A2  conjugate_a=off  conjugate_b=off  negate_abs=Normal  inmode_1_3=A*B  preaddmult_equ=A*B  preaddinsel=A  amultsel=A  bmultsel=B  inmode_0=A1  inmode_4=B1  logicinstr=X XOR Z  z_mux=0  xy_mux=P  w_mux=P  carry=CIN  operand=+  x_mux=P  XmcBlockStatus=1  maskContainerNames=tabcontainer1  block_type=opmode  block_config=sysgen:Opmode_config  block_height=1000
  Opmode1 : hdlBasic/Opmode  device=DSP58  equ=P=PCIN+(A*B)  operation=PCIN + A*B  inmode_0_3=D+A2  conjugate_a=off  conjugate_b=off  negate_abs=Negate  inmode_1_3=A*B  preaddmult_equ=-(A*B)  preaddinsel=A  amultsel=A  bmultsel=B  inmode_0=A2  inmode_4=B2  logicinstr=X XOR Z  z_mux=0  xy_mux=P  w_mux=P  carry=CIN  operand=+  x_mux=P  XmcBlockStatus=1  maskContainerNames=tabcontainer1  block_type=opmode  block_config=sysgen:Opmode_config  block_height=1000
  Opmode2 : hdlBasic/Opmode  device=DSP58  equ=P=(A*B)  operation=A * B  inmode_0_3=D+A2  conjugate_a=off  conjugate_b=off  negate_abs=Normal  inmode_1_3=A*B  preaddmult_equ=A*B  preaddinsel=A  amultsel=A  bmultsel=B  inmode_0=A1  inmode_4=B1  logicinstr=X XOR Z  z_mux=0  xy_mux=P  w_mux=P  carry=CIN  operand=+  x_mux=P  XmcBlockStatus=1  maskContainerNames=tabcontainer1  block_type=opmode  block_config=sysgen:Opmode_config  block_height=1000
  Opmode3 : hdlBasic/Opmode  device=DSP58  equ=P=PCIN+(A*B)  operation=PCIN + A*B  inmode_0_3=D+A2  conjugate_a=off  conjugate_b=off  negate_abs=Normal  inmode_1_3=A*B  preaddmult_equ=A*B  preaddinsel=A  amultsel=A  bmultsel=B  inmode_0=A2  inmode_4=B2  logicinstr=X XOR Z  z_mux=0  xy_mux=P  w_mux=P  carry=CIN  operand=+  x_mux=P  XmcBlockStatus=1  maskContainerNames=tabcontainer1  block_type=opmode  block_config=sysgen:Opmode_config  block_height=1000
  Terminator : Terminator
  Terminator1 : Terminator
  RE_O : Outport
  IM_O : Outport  Port=2
  tvalid_out : Outport  Port=3
  wires:
  Opmode/1 -> DSP58/3
  a_imag/1 -> DSP3/1, DSP1/1  "a_im"
  b_imag/1 -> DSP1/2, DSP2/2  "b_im"
  b_real/1 -> DSP3/2, DSP58/2  "b_re"
  a_real/1 -> DSP58/1, DSP2/1  "a_re"
  Opmode1/1 -> DSP1/4
  DSP58/2 -> DSP1/3
  Opmode2/1 -> DSP3/3
  Opmode3/1 -> DSP2/4
  DSP3/2 -> DSP2/3
  DSP1/1 -> RE_O/1
  DSP2/1 -> IM_O/1
  tvi_A/1 -> Logical/1  "a_re"
  Logical/1 -> tvalid_out/1
  tvi_B/1 -> Logical/2  "a_re"
  DSP58/1 -> Terminator/1
  DSP3/1 -> Terminator1/1
